simulink model "project2door"  (R2020b)
settings: Solver=VariableStepAuto  StartTime=0.0  StopTime=inf  RelTol=1e-3
settings Model: Creator=99003725  LastModifiedBy=99003725

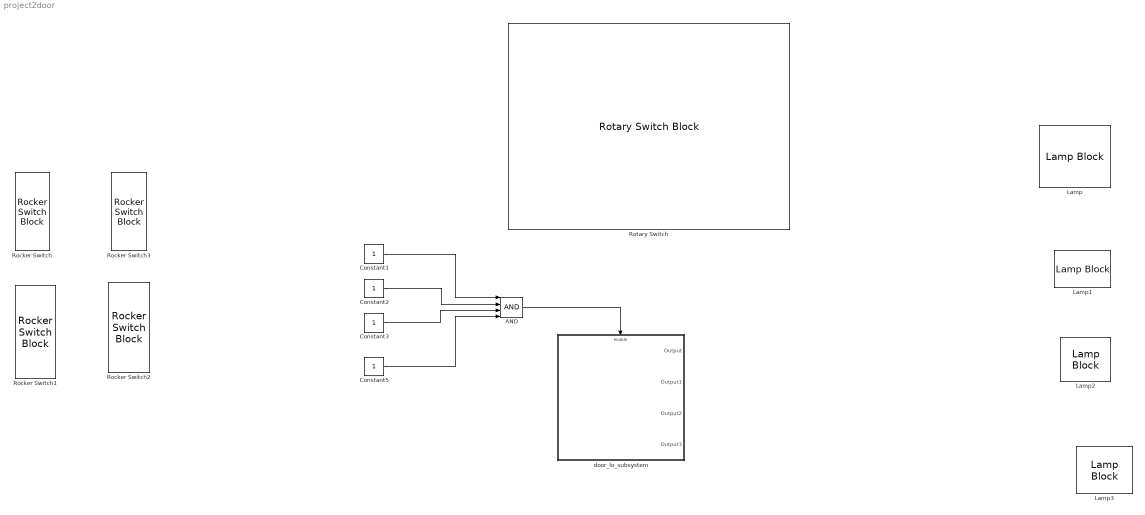
== system project2door ==
  AND : Logic  Inputs=4  IconShape=distinctive  AllPortsSameDT=off  OutDataTypeStr=boolean
  Constant{1..3,5} (4 alike) : Constant
  Lamp{,1..3} (4 alike) : LampBlock
  Rocker Switch{,1..3} (4 alike) : RockerSwitchBlock
      settings: Values={{'Off', 'On'}, [0 1]}
  Rotary Switch : RotarySwitchBlock
      settings: Values={{'automatic lock', 'lockoutpotetction', 'remote locking', 'delayed locking'}, [1 2 3 4]}
  door_lo_subsystem : Subsystem  TreatAsAtomicUnit=on
  wires:
  Constant3/1 -> AND/3
  Constant2/1 -> AND/2
  AND/1 -> door_lo_subsystem/Enable
  Constant5/1 -> AND/4
  Constant1/1 -> AND/1

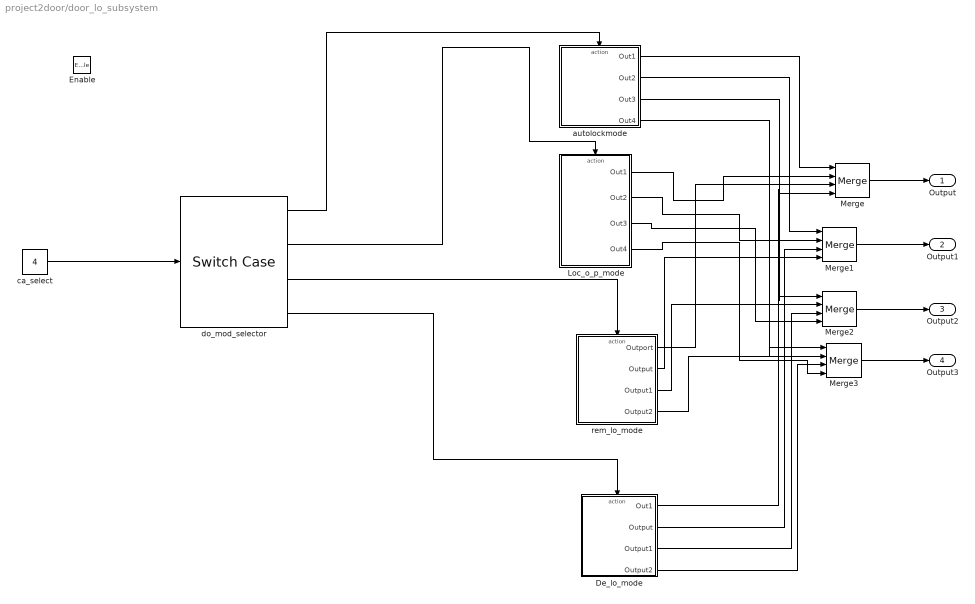
== system project2door/door_lo_subsystem ==
  Enable : EnablePort
  De_lo_mode : Subsystem  TreatAsAtomicUnit=on
  Loc_o_p_mode : Subsystem  TreatAsAtomicUnit=on
  Merge{,1..3} (4 alike) : Merge  Inputs=4
  autolockmode : Subsystem  TreatAsAtomicUnit=on
  ca_select : Constant  Value=4
  do_mod_selector : SwitchCase  CaseConditions={1,2,3,4}  ShowDefaultCase=off
  rem_lo_mode : Subsystem  TreatAsAtomicUnit=on
  Output : Outport
  Output1 : Outport  Port=2
  Output2 : Outport  Port=3
  Output3 : Outport  Port=4
  wires:
  ca_select/1 -> do_mod_selector/1
  do_mod_selector/3 -> rem_lo_mode/Action
  do_mod_selector/2 -> Loc_o_p_mode/Action
  do_mod_selector/1 -> autolockmode/Action
  autolockmode/1(Out1) -> Merge/1
  Loc_o_p_mode/1(Out1) -> Merge/2
  autolockmode/2(Out2) -> Merge1/1
  Loc_o_p_mode/2(Out2) -> Merge1/2
  autolockmode/3(Out3) -> Merge2/1
  Loc_o_p_mode/3(Out3) -> Merge2/4
  autolockmode/4(Out4) -> Merge3/1
  Loc_o_p_mode/4(Out4) -> Merge3/4
  rem_lo_mode/1(Outport) -> Merge/3
  rem_lo_mode/2(Output) -> Merge1/4
  rem_lo_mode/3(Output1) -> Merge2/2
  rem_lo_mode/4(Output2) -> Merge3/2
  Merge/1 -> Output/1
  Merge1/1 -> Output1/1
  Merge2/1 -> Output2/1
  Merge3/1 -> Output3/1
  do_mod_selector/4 -> De_lo_mode/Action
  De_lo_mode/1(Out1) -> Merge/4
  De_lo_mode/2(Output) -> Merge1/3
  De_lo_mode/3(Output1) -> Merge2/3
  De_lo_mode/4(Output2) -> Merge3/3

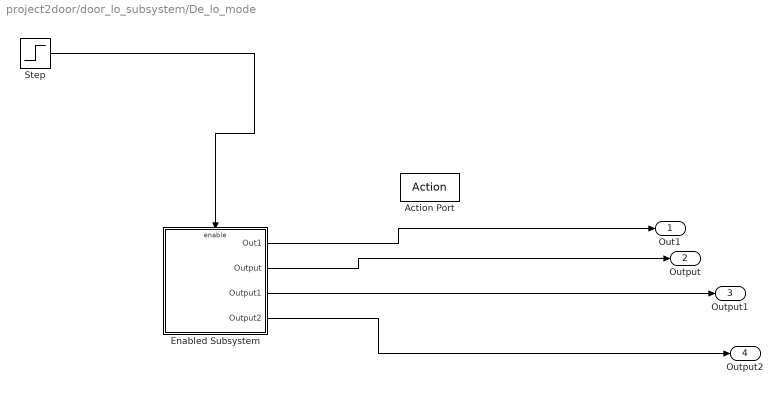
== system project2door/door_lo_subsystem/De_lo_mode ==
  Action Port : ActionPort  ActionPortLabel=case [ 4 ]:
  Enabled Subsystem : Subsystem  TreatAsAtomicUnit=on
  Step : Step  SampleTime=0
  Out1 : Outport
  Output : Outport  Port=2
  Output1 : Outport  Port=3
  Output2 : Outport  Port=4
  wires:
  Enabled Subsystem/1(Out1) -> Out1/1
  Step/1 -> Enabled Subsystem/Enable
  Enabled Subsystem/2(Output) -> Output/1
  Enabled Subsystem/3(Output1) -> Output1/1
  Enabled Subsystem/4(Output2) -> Output2/1

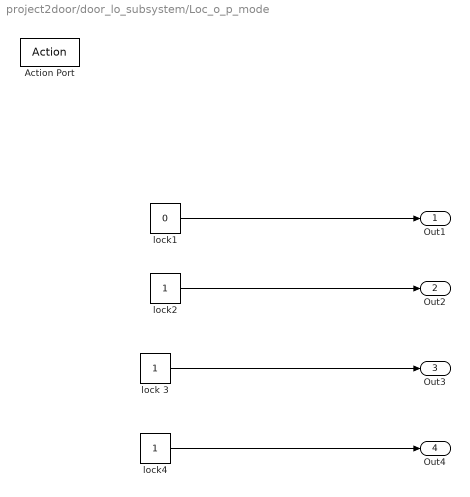
== system project2door/door_lo_subsystem/Loc_o_p_mode ==
  Action Port : ActionPort  ActionPortLabel=case [ 2 ]:
  lock 3 : Constant
  lock1 : Constant  Value=0
  lock2 : Constant
  lock4 : Constant
  Out1 : Outport
  Out2 : Outport  Port=2
  Out3 : Outport  Port=3
  Out4 : Outport  Port=4
  wires:
  lock2/1 -> Out2/1
  lock4/1 -> Out4/1
  lock 3/1 -> Out3/1
  lock1/1 -> Out1/1

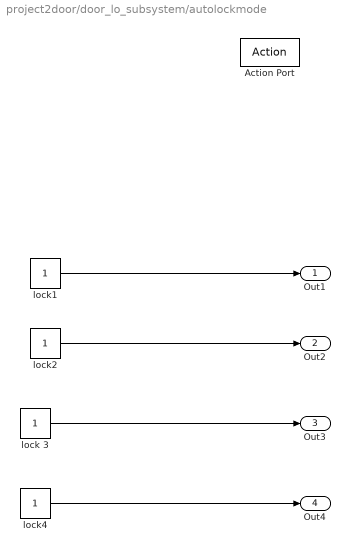
== system project2door/door_lo_subsystem/autolockmode ==
  Action Port : ActionPort  ActionPortLabel=case [ 1 ]:
  lock 3 : Constant
  lock1 : Constant
  lock2 : Constant
  lock4 : Constant
  Out1 : Outport
  Out2 : Outport  Port=2
  Out3 : Outport  Port=3
  Out4 : Outport  Port=4
  wires:
  lock 3/1 -> Out3/1
  lock2/1 -> Out2/1
  lock4/1 -> Out4/1
  lock1/1 -> Out1/1

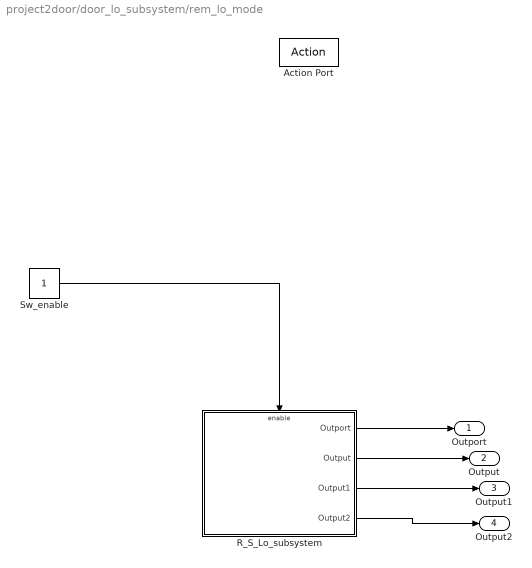
== system project2door/door_lo_subsystem/rem_lo_mode ==
  Action Port : ActionPort  ActionPortLabel=case [ 3 ]:
  R_S_Lo_subsystem : Subsystem  TreatAsAtomicUnit=on
  Sw_enable : Constant
  Outport : Outport
  Output : Outport  Port=2
  Output1 : Outport  Port=3
  Output2 : Outport  Port=4
  wires:
  Sw_enable/1 -> R_S_Lo_subsystem/Enable
  R_S_Lo_subsystem/1(Outport) -> Outport/1
  R_S_Lo_subsystem/2(Output) -> Output/1
  R_S_Lo_subsystem/3(Output1) -> Output1/1
  R_S_Lo_subsystem/4(Output2) -> Output2/1

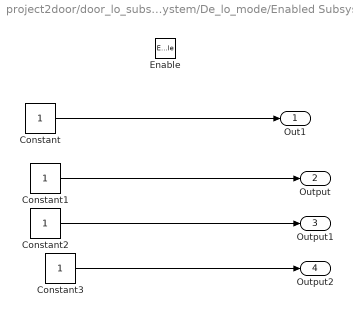
== system project2door/door_lo_subsystem/De_lo_mode/Enabled Subsystem ==
  Enable : EnablePort
  Constant{,1..3} (4 alike) : Constant
  Out1 : Outport
  Output : Outport  Port=2
  Output1 : Outport  Port=3
  Output2 : Outport  Port=4
  wires:
  Constant/1 -> Out1/1
  Constant1/1 -> Output/1
  Constant2/1 -> Output1/1
  Constant3/1 -> Output2/1

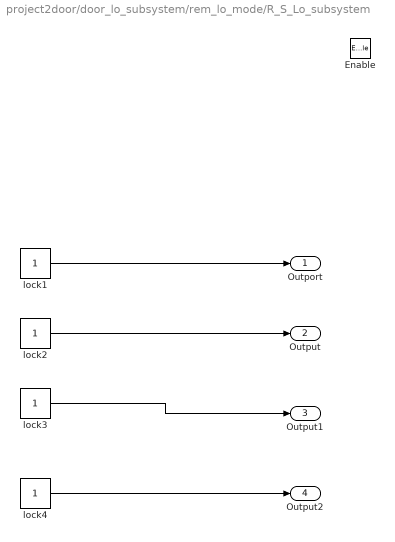
== system project2door/door_lo_subsystem/rem_lo_mode/R_S_Lo_subsystem ==
  Enable : EnablePort
  lock{1..4} (4 alike) : Constant
  Outport : Outport
  Output : Outport  Port=2
  Output1 : Outport  Port=3
  Output2 : Outport  Port=4
  wires:
  lock2/1 -> Output/1
  lock1/1 -> Outport/1
  lock4/1 -> Output2/1
  lock3/1 -> Output1/1
